simulink model "SPDynamicsWithDefinedInput"  (R2015a)
settings: Solver=ode45  StartTime=0.0  StopTime=10.0  RelTol=1e-3
settings Model: Creator=admin  LastModifiedBy=admin

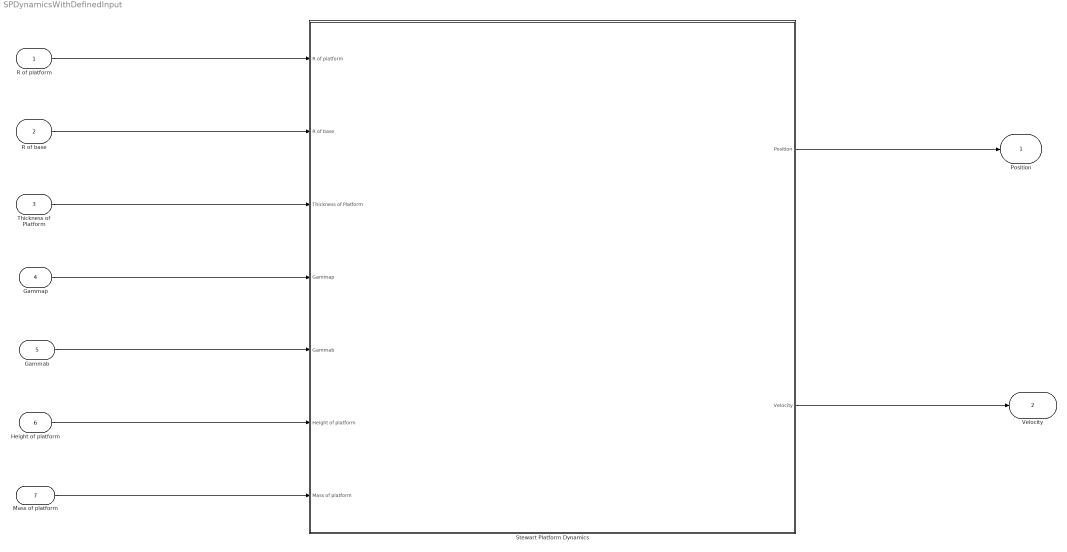
== system SPDynamicsWithDefinedInput ==
  R of platform : Inport
  R of base : Inport  Port=2
  Thickness of Platform : Inport  Port=3
  Gammap : Inport  Port=4
  Gammab : Inport  Port=5
  "Height of platform " : Inport  Port=6
  Mass of platform : Inport  Port=7
  Stewart Platform Dynamics : Subsystem
  Position : Outport
  Velocity : Outport  Port=2
  wires:
  R of platform/1 -> Stewart Platform Dynamics/1(R of platform)
  R of base/1 -> Stewart Platform Dynamics/2(R of base)
  Thickness of Platform/1 -> Stewart Platform Dynamics/3(Thickness of Platform)
  Gammap/1 -> Stewart Platform Dynamics/4(Gammap)
  Gammab/1 -> Stewart Platform Dynamics/5(Gammab)
  "Height of platform "/1 -> Stewart Platform Dynamics/6("Height of platform ")
  Mass of platform/1 -> Stewart Platform Dynamics/7(Mass of platform)
  Stewart Platform Dynamics/1(Position) -> Position/1
  Stewart Platform Dynamics/2(Velocity) -> Velocity/1

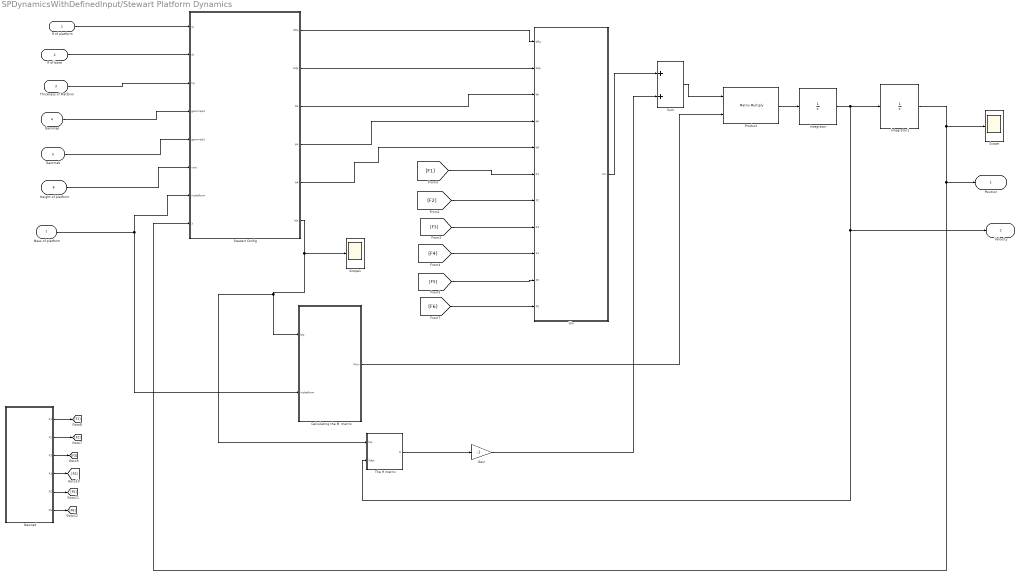
== system SPDynamicsWithDefinedInput/Stewart Platform Dynamics ==
  R of platform : Inport
  R of base : Inport  Port=2
  Thickness of Platform : Inport  Port=3
  Gammap : Inport  Port=4
  Gammab : Inport  Port=5
  "Height of platform " : Inport  Port=6
  Mass of platform : Inport  Port=7
  Calculating the M  matrix : MATLAB Function  TreatAsAtomicUnit=on
  Desired : Subsystem
  Gain : Gain  Gain=-1
  Integrator : Integrator
  Integrator1 : Integrator
  Product : Product  Multiplication=Matrix(*)
  Scope : Scope
  Scope1 : Scope
  Stewart Config : MATLAB Function  TreatAsAtomicUnit=on
  Sum : Sum  Inputs=|++
  The H matrix : MATLAB Function  TreatAsAtomicUnit=on
  Uin : MATLAB Function  TreatAsAtomicUnit=on
  Position : Outport
  Velocity : Outport  Port=2
  wires:
  Mass of platform/1 -> Calculating the M  matrix/2(mplatform), Stewart Config/7(mplatform)
  Stewart Config/3(bb) -> Uin/3(bb)
  Uin/1(Uin) -> Sum/1
  Stewart Config/2(bdp) -> Uin/2(bdp)
  Gain/1 -> Sum/2
  [F1] -> Uin/6(F1)
  [F2] -> Uin/7(F2)
  Gammap/1 -> Stewart Config/4(gammap1)
  [F3] -> Uin/8(F3)
  [F4] -> Uin/9(F4)
  Gammab/1 -> Stewart Config/5(gammab1)
  The H matrix/1(H) -> Gain/1
  Stewart Config/6(bIp) -> Scope1/1, Calculating the M  matrix/1(bIp), The H matrix/1(bIp)
  Stewart Config/5(bA) -> Uin/5(bA)
  Stewart Config/4(pp) -> Uin/4(pp)
  Integrator1/1 -> Stewart Config/8(X), Position/1, Scope/1
  Calculating the M  matrix/1(Minv) -> Product/2
  Sum/1 -> Product/1
  [F5] -> Uin/10(F5)
  [F6] -> Uin/11(F6)
  Product/1 -> Integrator/1
  R of platform/1 -> Stewart Config/1(rp)
  Integrator/1 -> Integrator1/1, The H matrix/2(Xdot), Velocity/1
  Thickness of Platform/1 -> Stewart Config/3(hp)
  "Height of platform "/1 -> Stewart Config/6(vert)
  R of base/1 -> Stewart Config/2(rb)
  Desired/1(F1) -> [F1]
  Desired/5(F5) -> [F5]
  Desired/4(F4) -> [F4]
  Desired/6(F6) -> [F6]
  Desired/2(F2) -> [F2]
  Desired/3(F3) -> [F3]
  Stewart Config/1(bRp) -> Uin/1(bRp)

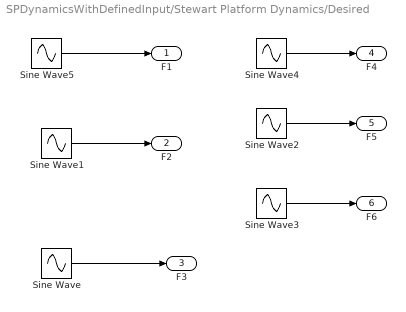
== system SPDynamicsWithDefinedInput/Stewart Platform Dynamics/Desired ==
  Sine Wave : Sin  Amplitude=0.29  Frequency=0.6283  SampleTime=0
  Sine Wave1 : Sin  Amplitude=0.3  Frequency=0.628  Phase=1.57  SampleTime=0
  Sine Wave2 : Sin  Amplitude=0.305  Frequency=0.6283  SampleTime=0
  Sine Wave3 : Sin  Amplitude=0.28  Frequency=0.6283  Phase=1.57  SampleTime=0
  Sine Wave4 : Sin  Amplitude=0.31  Frequency=0.6283  Phase=1.57  SampleTime=0
  Sine Wave5 : Sin  Amplitude=0.3  Frequency=0.628  SampleTime=0
  F1 : Outport
  F2 : Outport  Port=2
  F3 : Outport  Port=3
  F4 : Outport  Port=4
  F5 : Outport  Port=5
  F6 : Outport  Port=6
  wires:
  Sine Wave/1 -> F3/1
  Sine Wave1/1 -> F2/1
  Sine Wave5/1 -> F1/1
  Sine Wave2/1 -> F5/1
  Sine Wave3/1 -> F6/1
  Sine Wave4/1 -> F4/1

== matlab function SPDynamicsWithDefinedInput/Stewart Platform Dynamics/Stewart Config ==
  data: rp input; bRp output; rb input; hp input; gammap1 input; gammab1 input; vert input; mplatform input; X input; bdp output; bb output; pp output; bA output; bIp output
function [bRp,bdp,bb,pp,bA,bIp] = fcn(rp,rb,hp,gammap1,gammab1,vert,mplatform,X)
%#codegen
%The states that were chosen were X=[x,y,z,phi,theta,psi] and
%X2=[xdot,ydot,zdot,p,q,r ]
%Due to this a  trnasformation matrix must be added to transform the body
%rates to Euler rates.
gammap = [gammap1,120-gammap1, 120+gammap1, -120-gammap1,-120+gammap1,-gammap1];
gammab = [gammab1,120-gammab1, 120+gammab1, -120-gammab1,-120+gammab1,-gammab1];

 %alphap = [0 , 120, 120, -120 , -120 , 0] ;  
 %betab = [60,60,180,180,-60,-60];
 
 
 % pIp = mplatform *[((rp^2)/4) , 0, 0; 0, ((rp*2)/4), 0; 0, 0, (rp^2)/2] ;
    pp=zeros(3,6);
    pp(1,: ) = rp*cos(gammap*pi/180);
    pp(2,: ) = rp*sin(gammap*pi/180) ;
    pp(3,: ) = [hp/2,hp/2,hp/2,hp/2,hp/2,hp/2 ] ;        %hp is the thickness of the platform
    bb=zeros(3,6);
    bb(1,: ) = rb*cos(gammab*pi/180);
    bb(2,: ) = rb*sin(gammab*pi/180);
    bb(3,: ) = [0 , 0, 0, 0 , 0, 0] ;
    
     bdp = [X(1,a),X(2,a),X(3,a)+vert]' ;                        %Position of platform frame wrt base
    bDp = [bdp,bdp,bdp,bdp,bdp,bdp] ;                           %This is same for all 6 actuators
   
      psi=X(4,a);
      the=X(5,a);
      phi=X(6,a);
    
   
    spsi = sin(psi);
    cpsi = cos(psi);
    sthe = sin(the);
    cthe = cos(the);
    sphi = sin(phi);
    cphi = cos(phi);
    
    
    pIp = mplatform *[((0.15^2)/4) , 0, 0; 0, ((0.15*2)/4), 0; 0, 0, (0.15^2)/2] ;
    bRp=zeros(3,3);
    bRp(1,1 ) = cphi * cthe ;
    bRp(1,2 ) = -sphi*cpsi + cphi * sthe * spsi ;
    bRp(1,3 ) = sphi * spsi + cphi * sthe * cpsi ;
    bRp(2,1 ) = sphi * cthe ;
    bRp(2,2 ) = cphi * cpsi + sphi * sthe * spsi ;
    bRp(2,3 ) = -cphi * spsi + sphi * sthe * cpsi ;
    bRp(3,1 ) = -sthe ;
    bRp(3,2 ) = cthe * spsi ;
    bRp(3,3 ) = cthe * cpsi ;
    
     bA = bRp*pp + bDp - bb ;                                    %Actuator vector
    
     bIp=bRp*pIp*bRp';                                           %Inertia tensor varying due to orientation of platform wrt base

== matlab function SPDynamicsWithDefinedInput/Stewart Platform Dynamics/Uin ==
  data: bRp input; bdp input; bb input; Uin output; pp input; bA input; F1 input; F2 input; F3 input; F4 input; F5 input; F6 input
function Uin = fcn(bRp,bdp,bb,pp,bA,F1,F2,F3,F4,F5,F6)
%#codegen
    g=9.81;
    G=[0,0,-g]';
    Fvec=zeros(3,6);
    %We are going to add g in vector form to the input force
   
    %for j=1:6
     %  Fvec(:,j)=F(j,a)*bA(:,j);
    %end
    Fvec(:,1)=F1*bA(:,1);
    Fvec(:,2)=F2*bA(:,2);
    Fvec(:,3)=F3*bA(:,3);
    Fvec(:,4)=F4*bA(:,4);
    Fvec(:,5)=F5*bA(:,5);
    Fvec(:,6)=F6*bA(:,6);
      
    
   U=zeros(6,1);                                              %Combined effect of gravity and force on actuators
     %for j=1:6
      % U(j,1)= F(j,a)+dot(Fvec(:,j),G);
     %end
     
     
     U(1,1)=F1+dot(Fvec(:,1),G);
     U(2,1)=F2+dot(Fvec(:,2),G);
     U(3,1)=F3+dot(Fvec(:,3),G);
     U(4,1)=F4+dot(Fvec(:,4),G);
     U(5,1)=F5+dot(Fvec(:,5),G);
     U(6,1)=F6+dot(Fvec(:,6),G);
    
     Jt=zeros(6,6);
   
      for i=1:6
      Jt(:,i ) = [ ( bRp*pp(:,i) + bdp - bb(:,i) ); cross( bRp*pp(:,i),bdp-bb(:,i) ) ] / norm(bA(:,i)) ;
  
      end
    
     Uin=Jt*U;                                                %Input u in state space form

== matlab function SPDynamicsWithDefinedInput/Stewart Platform Dynamics/Calculating the M  matrix ==
  data: bIp input; mplatform input; Minv output
function Minv = fcn(bIp,mplatform)
%#codegen
Minv=zeros(6,6);
m=mplatform*(eye(3));

z=zeros(3,3);

M=[m,z;z,bIp];
Minv=inv(M);

== matlab function SPDynamicsWithDefinedInput/Stewart Platform Dynamics/The H matrix ==
  data: bIp input; H output; Xdot input
function H = fcn(bIp,Xdot)
%#codegen

bWp = [Xdot(4,1) ; Xdot(5,1) ; Xdot(6,1)] ;

bWpskew=[ 0 , -1*bWp(3,1) , bWp(2,1) ; 
         bWp(3,1) , 0 , -1*bWp(1,1)  ;
         -1*bWp(2,1), bWp(1,1), 0 ];
     
     h= bWpskew*bIp;                             %WxI 
    H=[z,z;z,h];
